simulink library "usask_segmented_TLM_lib"  (R2018a)
settings: Solver=VariableStepAuto  StartTime=0.0  StopTime=10.0  RelTol=1e-3
values from neighbouring files (symbols this model uses):
  beta = [1e-05 1.21547425008e-05 1.4773776526e-05 1.79571449437e-05 2.1826447284e-05 2.65294846443e-05 3.2245905453e-05 3.91940677485e-05 4.7639380104e-05 5.7904439806e-05 7.03813555493e-05 8.55467253557e-05 ... (60 elements, 1x60)]    [G_lookup.mat]    (also in H_lookup.mat)
  lambda_A = [0.333333333333 0.351351351351 0.369863013699 0.388888888889 0.408450704225 0.428571428571 0.449275362319 0.470588235294 0.492537313433 0.515151515152 0.538461538462 0.5625 ... (51 elements, 1x51)]    [H_lookup.mat]
  n = [6 3 2 1.5 1.2 1]    [G_lookup.mat]    (also in interpolate_G.m = lu_data.n)
  n1 = [0 16.6666666667 8.33333333333 5.55555555556 4.16666666667 3.33333333333]    [H_lookup.mat]    (also in interpolate_H.m = lu_data.n1)
  n2 = [0 16.6666666667 8.33333333333 5.55555555556 4.16666666667 3.33333333333]    [H_lookup.mat]    (also in interpolate_H.m = lu_data.n2)
  n3 = [3.16296285985 3.12622720794 3.08950324161 3.03556206993 2.98109456935 2.92539200093 2.86604767633 2.80095613668 2.7359041708 2.66771255902 2.60605912149 2.43399666463 ... (3060 elements, 60x51)]    [H_lookup.mat]    (also in interpolate_H.m = interp2(lu_data.phi_A,log10(lu_data.beta),lu_data.n3,phi,log)
  W1 = [0.817804106601 -0.379201060736 4.74543844452 -19.7629025979 31.2965927958 -16.3931724883 0.817756661365 -0.379072651507 4.74402355955 -19.7576226526 31.2889826509 -16.3894979768 ... (18360 elements, 1x6x60x51)]    [H_lookup.mat]    (also in interpolate_H.m = nan(size(n1)))
  W2 = [-0.0342032638777 0.250736765493 -2.89749565946 11.0980283604 -15.789942854 7.03898081697 -0.034202667139 0.250724810196 -2.89736972734 11.0975869151 -15.789368559 7.03873652617 ... (18360 elements, 1x6x60x51)]    [H_lookup.mat]    (also in interpolate_H.m = nan(size(n2)))
  W3 = H_DC3*n3/2    [interpolate_H.m]
undefined symbols (not defined in the file or in its folder): K, L, m_G, nu, rA, rB, rho, T, Zc_A, Zc_B
libraries: $bdroot x34
settings Model: Creator=tkw954  LastModifiedBy=tkw954

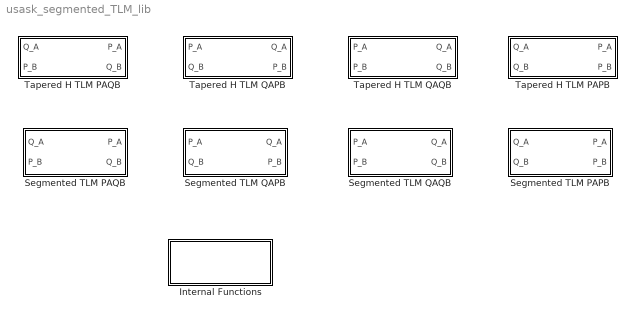
== system usask_segmented_TLM_lib ==
  Internal Functions : Subsystem
  Segmented TLM PAPB : Subsystem  mask{x_LU=100*[0 0.5 1], d_LU=12e-3*[1 0.8 1], K=1e6, nu=100e-6, rho=850}
      mask prompts: x_LU "Shape Lookup Lengths (m)"; d_LU "Shape Lookup Diameters (m)"; K "Oil Bulk Modulus (Pa)"; nu "Oil Viscosity (m^2/s)"; rho "Oil Density (kg/m^3)"
      mask init:
      | if numel(x_LU)~=numel(d_LU)
      |     error('size of x lookup table must be same as d lookup table')
      | end
      | 
      | 
      | dx = 120;
      | y = 30;
      | w_seg = 70;
      | %w_min=30;
      | %w_space=20;
      | h = 100;
      | 
      | x_LU=x_LU-x_LU(1);%ensure first point is 0
      | 
      | N=numel(x_LU)-1;%number of segments
      | 
      | %model parameters
      | 
      | c=sqrt(K/rho);
      | Zc=rho*c./(pi/4*d_LU.^2);
      | Zc_A=Zc(1);
      | Zc_B=Zc(end);
      | 
      | delta_x=diff(x_LU);
      | T=delta_x/c
      | 
      | lambda_A=d_LU(2:end)./d_LU(1:(end-1))
      | 
      | beta = ((nu*delta_x)./(c*(d_LU(1:(end-1))/2).^2)).*((lambda_A.^2+lambda_A+1).^2./(9*lambda_A.^3)) % Dissipation number (dimensionless)
      | 
      | % 
      | % %find and delete old blocks and lines
      | sys=gcb;
      | hcb=get_param(sys,'Handle');
      | hb=get(hcb,'blocks');
      | segment_name='segment';
      | idx_seg=find(strncmp(hb,segment_name,numel(segment_name)));%find segments
      | assignin('base','hb',hb)
      | assignin('base','hcb',hcb)
      | assignin('base','idx_seg',idx_seg)
      | 
      | for i=1:numel(idx_seg)
      |     delete_block(sprintf('%s/%s',sys, hb{idx_seg(i)}))
      | end
      | 
      | hlines=get(hcb,'lines');
      | for i=1:numel(hlines)
      |     delete_line(hlines(i).Handle)
      | end
      | 
      | for i=1:N
      |     pos = [dx*i y dx*i+w_seg y+h];
      |     add_block('usask_segmented_TLM_lib/Internal Functions/Tapered TLM Segment',sprintf('%s/%s_%d',sys,segment_name, i),'Position',pos);
      |       set_param(sprintf('%s/%s_%d',sys,segment_name, i),'beta',sprintf('beta(%d)',i));
      |           set_param(sprintf('%s/%s_%d',sys,segment_name, i),'T',sprintf('T(%d)',i));
      |           set_param(sprintf('%s/%s_%d',sys,segment_name, i),'lambda_A',sprintf('lambda_A(%d)',i));
      | 
      | 
      | end
      | % 
      | % 
      | 
      | add_line(sys,'Q_A/1','Boundary A/1','autorouting','on')
      | add_line(sys,'Boundary A/1','P_A/1','autorouting','on')
      | add_line(sys,'Q_B/1','Boundary B/1','autorouting','on')
      | add_line(sys,'Boundary B/1','P_B/1','autorouting','on')
      | 
      | add_line(sys,'Boundary A/2','segment_1/1','autorouting','on')
      | add_line(sys,'segment_1/1','Boundary A/2','autorouting','on')
      | 
      | add_line(sys,'Boundary B/2',sprintf('%s_%d/2',segment_name, N),'autorouting','on')
      | add_line(sys,sprintf('%s_%d/2',segment_name, N),'Boundary B/2','autorouting','on')
      | 
      | for i=1:(N-1)
      |     add_line(sys,sprintf('segment_%d/2',i),sprintf('segment_%d/1',i+1),'autorouting','on')
      |      add_line(sys,sprintf('segment_%d/1',i+1),sprintf('segment_%d/2',i),'autorouting','on')
      |    
      | end
      mask Display:
      | port_label('input', 1 , '\itq_A', 'texmode', 'on')
      | port_label('input', 2 , '\itq_B', 'texmode', 'on')
      | port_label('output', 1 , '\itp_A', 'texmode', 'on')
      | port_label('output', 2 , '\itp_B', 'texmode', 'on')
      | 
      | plot(x_LU,d_LU)
      | plot(x_LU,-d_LU)
  Segmented TLM PAQB : Subsystem  mask{x_LU=100*[0 0.5 1], d_LU=12e-3*[1 0.8 1], K=1e6, nu=100e-6, rho=850}
      mask prompts: x_LU "Shape Lookup Lengths (m)"; d_LU "Shape Lookup Diameters (m)"; K "Oil Bulk Modulus (Pa)"; nu "Oil Viscosity (m^2/s)"; rho "Oil Density (kg/m^3)"
      mask init:
      | if numel(x_LU)~=numel(d_LU)
      |     error('size of x lookup table must be same as d lookup table')
      | end
      | 
      | 
      | dx = 120;
      | y = 30;
      | w_seg = 70;
      | %w_min=30;
      | %w_space=20;
      | h = 100;
      | 
      | x_LU=x_LU-x_LU(1);%ensure first point is 0
      | 
      | N=numel(x_LU)-1;%number of segments
      | 
      | %model parameters
      | 
      | c=sqrt(K/rho);
      | Zc=rho*c./(pi/4*d_LU.^2);
      | Zc_A=Zc(1);
      | Zc_B=Zc(end);
      | 
      | delta_x=diff(x_LU);
      | T=delta_x/c
      | 
      | lambda_A=d_LU(2:end)./d_LU(1:(end-1))
      | 
      | beta = ((nu*delta_x)./(c*(d_LU(1:(end-1))/2).^2)).*((lambda_A.^2+lambda_A+1).^2./(9*lambda_A.^3)) % Dissipation number (dimensionless)
      | 
      | % 
      | % %find and delete old blocks and lines
      | sys=gcb;
      | hcb=get_param(sys,'Handle');
      | hb=get(hcb,'blocks');
      | segment_name='segment';
      | idx_seg=find(strncmp(hb,segment_name,numel(segment_name)));%find segments
      | assignin('base','hb',hb)
      | assignin('base','hcb',hcb)
      | assignin('base','idx_seg',idx_seg)
      | 
      | for i=1:numel(idx_seg)
      |     delete_block(sprintf('%s/%s',sys, hb{idx_seg(i)}))
      | end
      | 
      | hlines=get(hcb,'lines');
      | for i=1:numel(hlines)
      |     delete_line(hlines(i).Handle)
      | end
      | 
      | for i=1:N
      |     pos = [dx*i y dx*i+w_seg y+h];
      |     add_block('usask_segmented_TLM_lib/Internal Functions/Tapered TLM Segment',sprintf('%s/%s_%d',sys,segment_name, i),'Position',pos);
      |       set_param(sprintf('%s/%s_%d',sys,segment_name, i),'beta',sprintf('beta(%d)',i));
      |           set_param(sprintf('%s/%s_%d',sys,segment_name, i),'T',sprintf('T(%d)',i));
      |           set_param(sprintf('%s/%s_%d',sys,segment_name, i),'lambda_A',sprintf('lambda_A(%d)',i));
      | 
      | 
      | end
      | % 
      | % 
      | 
      | add_line(sys,'Q_A/1','Boundary A/1','autorouting','on')
      | add_line(sys,'Boundary A/1','P_A/1','autorouting','on')
      | add_line(sys,'P_B/1','Boundary B/1','autorouting','on')
      | add_line(sys,'Boundary B/1','Q_B/1','autorouting','on')
      | 
      | add_line(sys,'Boundary A/2','segment_1/1','autorouting','on')
      | add_line(sys,'segment_1/1','Boundary A/2','autorouting','on')
      | 
      | add_line(sys,'Boundary B/2',sprintf('%s_%d/2',segment_name, N),'autorouting','on')
      | add_line(sys,sprintf('%s_%d/2',segment_name, N),'Boundary B/2','autorouting','on')
      | 
      | for i=1:(N-1)
      |     add_line(sys,sprintf('segment_%d/2',i),sprintf('segment_%d/1',i+1),'autorouting','on')
      |      add_line(sys,sprintf('segment_%d/1',i+1),sprintf('segment_%d/2',i),'autorouting','on')
      |    
      | end
      mask Display:
      | port_label('input', 1 , '\itq_A', 'texmode', 'on')
      | port_label('input', 2 , '\itp_B', 'texmode', 'on')
      | port_label('output', 1 , '\itp_A', 'texmode', 'on')
      | port_label('output', 2 , '\itq_B', 'texmode', 'on')
      | 
      | plot(x_LU,d_LU)
      | plot(x_LU,-d_LU)
  Segmented TLM QAPB : Subsystem  mask{x_LU=100*[0 0.5 1], d_LU=12e-3*[1 0.8 1], K=1e9, nu=100e-6, rho=850}
      mask prompts: x_LU "Shape Lookup Lengths (m)"; d_LU "Shape Lookup Diameters (m)"; K "Oil Bulk Modulus (Pa)"; nu "Oil Viscosity (m^2/s)"; rho "Oil Density (kg/m^3)"
      mask init:
      | if numel(x_LU)~=numel(d_LU)
      |     error('size of x lookup table must be same as d lookup table')
      | end
      | 
      | 
      | dx = 120;
      | y = 30;
      | w_seg = 70;
      | %w_min=30;
      | %w_space=20;
      | h = 100;
      | 
      | x_LU=x_LU-x_LU(1);%ensure first point is 0
      | 
      | N=numel(x_LU)-1;%number of segments
      | 
      | %model parameters
      | 
      | c=sqrt(K/rho);
      | Zc=rho*c./(pi/4*d_LU.^2);
      | Zc_A=Zc(1);
      | Zc_B=Zc(end);
      | 
      | delta_x=diff(x_LU);
      | T=delta_x/c
      | 
      | lambda_A=d_LU(2:end)./d_LU(1:(end-1))
      | 
      | beta = ((nu*delta_x)./(c*(d_LU(1:(end-1))/2).^2)).*((lambda_A.^2+lambda_A+1).^2./(9*lambda_A.^3)) % Dissipation number (dimensionless)
      | 
      | % 
      | % %find and delete old blocks and lines
      | sys=gcb;
      | hcb=get_param(sys,'Handle');
      | hb=get(hcb,'blocks');
      | segment_name='segment';
      | idx_seg=find(strncmp(hb,segment_name,numel(segment_name)));%find segments
      | assignin('base','hb',hb)
      | assignin('base','hcb',hcb)
      | assignin('base','idx_seg',idx_seg)
      | 
      | for i=1:numel(idx_seg)
      |     delete_block(sprintf('%s/%s',sys, hb{idx_seg(i)}))
      | end
      | 
      | hlines=get(hcb,'lines');
      | for i=1:numel(hlines)
      |     delete_line(hlines(i).Handle)
      | end
      | 
      | for i=1:N
      |     pos = [dx*i y dx*i+w_seg y+h];
      |     add_block('usask_segmented_TLM_lib/Internal Functions/Tapered TLM Segment',sprintf('%s/%s_%d',sys,segment_name, i),'Position',pos);
      |       set_param(sprintf('%s/%s_%d',sys,segment_name, i),'beta',sprintf('beta(%d)',i));
      |           set_param(sprintf('%s/%s_%d',sys,segment_name, i),'T',sprintf('T(%d)',i));
      |           set_param(sprintf('%s/%s_%d',sys,segment_name, i),'lambda_A',sprintf('lambda_A(%d)',i));
      | 
      | 
      | end
      | % 
      | % 
      | 
      | add_line(sys,'P_A/1','Boundary A/1','autorouting','on')
      | add_line(sys,'Boundary A/1','Q_A/1','autorouting','on')
      | add_line(sys,'Q_B/1','Boundary B/1','autorouting','on')
      | add_line(sys,'Boundary B/1','P_B/1','autorouting','on')
      | 
      | add_line(sys,'Boundary A/2','segment_1/1','autorouting','on')
      | add_line(sys,'segment_1/1','Boundary A/2','autorouting','on')
      | 
      | add_line(sys,'Boundary B/2',sprintf('%s_%d/2',segment_name, N),'autorouting','on')
      | add_line(sys,sprintf('%s_%d/2',segment_name, N),'Boundary B/2','autorouting','on')
      | 
      | for i=1:(N-1)
      |     add_line(sys,sprintf('segment_%d/2',i),sprintf('segment_%d/1',i+1),'autorouting','on')
      |      add_line(sys,sprintf('segment_%d/1',i+1),sprintf('segment_%d/2',i),'autorouting','on')
      |    
      | end
      mask Display:
      | port_label('input', 1 , '\itp_A', 'texmode', 'on')
      | port_label('input', 2 , '\itq_B', 'texmode', 'on')
      | port_label('output', 1 , '\itq_A', 'texmode', 'on')
      | port_label('output', 2 , '\itp_B', 'texmode', 'on')
      | 
      | plot(x_LU,d_LU)
      | plot(x_LU,-d_LU)
  Segmented TLM QAQB : Subsystem  mask{x_LU=100*[0 0.5 1], d_LU=12e-3*[1 0.8 1], K=1e9, nu=100e-6, rho=850}
      mask prompts: x_LU "Shape Lookup Lengths (m)"; d_LU "Shape Lookup Diameters (m)"; K "Oil Bulk Modulus (Pa)"; nu "Oil Viscosity (m^2/s)"; rho "Oil Density (kg/m^3)"
      mask init:
      | if numel(x_LU)~=numel(d_LU)
      |     error('size of x lookup table must be same as d lookup table')
      | end
      | 
      | 
      | dx = 120;
      | y = 30;
      | w_seg = 70;
      | %w_min=30;
      | %w_space=20;
      | h = 100;
      | 
      | x_LU=x_LU-x_LU(1);%ensure first point is 0
      | 
      | lambda_A=d_LU(2:end)./d_LU(1:(end-1));
      | 
      | phi=(lambda_A-1)./(lambda_A+1);
      | 
      | phi_max=0.5;
      | 
      | while any(abs(phi)>phi_max)
      |     idx=find(abs(phi)>phi_max,1);
      |     d_LU=[d_LU(1:idx) (d_LU(idx)+d_LU(idx+1))/2 d_LU((idx+1):end)];
      |     x_LU=[x_LU(1:idx) (x_LU(idx)+x_LU(idx+1))/2 x_LU((idx+1):end)];
      |     lambda_A=d_LU(2:end)./d_LU(1:(end-1));
      | 
      |     phi=(lambda_A-1)./(lambda_A+1);
      | end
      | 
      | 
      | N=numel(x_LU)-1;%number of segments
      | 
      | %model parameters
      | 
      | c=sqrt(K/rho);
      | Zc=rho*c./(pi/4*d_LU.^2);
      | Zc_A=Zc(1);
      | Zc_B=Zc(end);
      | 
      | delta_x=diff(x_LU);
      | T=delta_x/c
      | 
      | 
      | 
      | beta = ((nu*delta_x)./(c*(d_LU(1:(end-1))/2).^2)).*((lambda_A.^2+lambda_A+1).^2./(9*lambda_A.^3)) % Dissipation number (dimensionless)
      | lambda_A
      | 
      | % 
      | % %find and delete old blocks and lines
      | sys=gcb;
      | hcb=get_param(sys,'Handle');
      | hb=get(hcb,'blocks');
      | segment_name='segment';
      | idx_seg=find(strncmp(hb,segment_name,numel(segment_name)));%find segments
      | assignin('base','hb',hb)
      | assignin('base','hcb',hcb)
      | assignin('base','idx_seg',idx_seg)
      | 
      | for i=1:numel(idx_seg)
      |     delete_block(sprintf('%s/%s',sys, hb{idx_seg(i)}))
      | end
      | 
      | hlines=get(hcb,'lines');
      | for i=1:numel(hlines)
      |     delete_line(hlines(i).Handle)
      | end
      | 
      | for i=1:N
      |     pos = [dx*i y dx*i+w_seg y+h];
      |     add_block('usask_segmented_TLM_lib/Internal Functions/Tapered TLM Segment',sprintf('%s/%s_%d',sys,segment_name, i),'Position',pos);
      |       set_param(sprintf('%s/%s_%d',sys,segment_name, i),'beta',sprintf('beta(%d)',i));
      |           set_param(sprintf('%s/%s_%d',sys,segment_name, i),'T',sprintf('T(%d)',i));
      |           set_param(sprintf('%s/%s_%d',sys,segment_name, i),'lambda_A',sprintf('lambda_A(%d)',i));
      | 
      | 
      | end
      | % 
      | % 
      | 
      | add_line(sys,'P_A/1','Boundary A/1','autorouting','on')
      | add_line(sys,'Boundary A/1','Q_A/1','autorouting','on')
      | add_line(sys,'P_B/1','Boundary B/1','autorouting','on')
      | add_line(sys,'Boundary B/1','Q_B/1','autorouting','on')
      | 
      | add_line(sys,'Boundary A/2','segment_1/1','autorouting','on')
      | add_line(sys,'segment_1/1','Boundary A/2','autorouting','on')
      | 
      | add_line(sys,'Boundary B/2',sprintf('%s_%d/2',segment_name, N),'autorouting','on')
      | add_line(sys,sprintf('%s_%d/2',segment_name, N),'Boundary B/2','autorouting','on')
      | 
      | for i=1:(N-1)
      |     add_line(sys,sprintf('segment_%d/2',i),sprintf('segment_%d/1',i+1),'autorouting','on')
      |      add_line(sys,sprintf('segment_%d/1',i+1),sprintf('segment_%d/2',i),'autorouting','on')
      |    
      | end
      mask Display:
      | port_label('input', 1 , '\itp_A', 'texmode', 'on')
      | port_label('input', 2 , '\itp_B', 'texmode', 'on')
      | port_label('output', 1 , '\itq_A', 'texmode', 'on')
      | port_label('output', 2 , '\itq_B', 'texmode', 'on')
      | 
      | plot(x_LU,d_LU)
      | plot(x_LU,-d_LU)
  Tapered H TLM PAPB : Subsystem  mask(Tapered Hydraulic Transmission Line (TLM)){D_A=rA*2, D_B=rB*2, L=L, K=K, nu=nu, rho=rho}
      mask prompts: D_A "Inlet Diameter (m)"; D_B "Outlet Diameter (m)"; L "Length (m)"; K "Oil Bulk Modulus (Pa)"; nu "Oil Viscosity (m^2/s)"; rho "Oil Density (kg/m^3)"
      mask help:
      | This model implements the transmission line model in Wiens and ven der Buhs (2018).
      |
      | This model assumes a rigid-walled tube with a linear taper in radius between the two ports. It assumes constant bulk modulus (no cavitation or entrained air effects) and includes frequency-dependent friction effects.
      |
      | Positive flows are directed into either port.
      |
      | This model also assumes zero initial conditions
      |
      | Reference:
      | Travis Wiens and Jeremy vsn der Buhs. Transmission Line Modelling of Laminar Liquid Wave Propagation in Tapered Tubes. In preparation.
      mask init:
      | % Check for positive params, report error if negative given
      | if D_A<0 || D_B<0 || L<0 || K<0 || nu<0 || rho<0
      |     error('Please ensure parameters are all positive')
      | end
      | 
      | r_A = D_A/2; % Inlet radius (m)
      | r_B = D_B/2; % Outlet radius (m)
      | 
      | c=sqrt(K/rho);% Local speed of sound (m/s)
      | lambda_A = r_B/r_A; % Taper ratio (dimensionless)
      | beta = ((nu*L)/(c*r_A^2))*((lambda_A^2+lambda_A+1)^2/(9*lambda_A^3)); % Dissipation number (dimensionless)
      | Zc_A=c*rho/(pi*r_A^2);
      | Zc_B=c*rho/(pi*r_B^2);
      | T=L/c; % Wave propagation time (s)
      mask DialogControl DescGroupVar Prompt: Tapered Hydraulic Transmission Line (TLM)
      mask Display:
      | port_label('input', 1 , '\itq_A', 'texmode', 'on')
      | port_label('input', 2 , '\itq_B', 'texmode', 'on')
      | port_label('output', 1 , '\itp_A', 'texmode', 'on')
      | port_label('output', 2 , '\itp_B', 'texmode', 'on')
  Tapered H TLM PAQB : Subsystem  mask(Tapered Hydraulic Transmission Line (TLM)){D_A=rA*2, D_B=rB*2, L=L, K=K, nu=nu, rho=rho}
      mask prompts: D_A "Inlet Diameter (m)"; D_B "Outlet Diameter (m)"; L "Length (m)"; K "Oil Bulk Modulus (Pa)"; nu "Oil Viscosity (m^2/s)"; rho "Oil Density (kg/m^3)"
      mask help:
      | This model implements the transmission line model in Wiens and ven der Buhs (2018).
      |
      | This model assumes a rigid-walled tube with a linear taper in radius between the two ports. It assumes constant bulk modulus (no cavitation or entrained air effects) and includes frequency-dependent friction effects.
      |
      | Positive flows are directed into either port.
      |
      | This model also assumes zero initial conditions
      |
      | Reference:
      | Travis Wiens and Jeremy vsn der Buhs. Transmission Line Modelling of Laminar Liquid Wave Propagation in Tapered Tubes. In preparation.
      mask init:
      | % Check for positive params, report error if negative given
      | if D_A<0 || D_B<0 || L<0 || K<0 || nu<0 || rho<0
      |     error('Please ensure parameters are all positive')
      | end
      | 
      | r_A = D_A/2; % Inlet radius (m)
      | r_B = D_B/2; % Outlet radius (m)
      | 
      | c=sqrt(K/rho);% Local speed of sound (m/s)
      | lambda_A = r_B/r_A; % Taper ratio (dimensionless)
      | beta = ((nu*L)/(c*r_A^2))*((lambda_A^2+lambda_A+1)^2/(9*lambda_A^3)); % Dissipation number (dimensionless)
      | Zc_A=c*rho/(pi*r_A^2);
      | Zc_B=c*rho/(pi*r_B^2);
      | T=L/c; % Wave propagation time (s)
      mask DialogControl DescGroupVar Prompt: Tapered Hydraulic Transmission Line (TLM)
      mask Display:
      | port_label('input', 1 , '\itq_A', 'texmode', 'on')
      | port_label('input', 2 , '\itp_B', 'texmode', 'on')
      | port_label('output', 1 , '\itp_A', 'texmode', 'on')
      | port_label('output', 2 , '\itq_B', 'texmode', 'on')
  Tapered H TLM QAPB : Subsystem  mask(Tapered Hydraulic Transmission Line (TLM)){D_A=rA*2, D_B=rB*2, L=L, K=K, nu=nu, rho=rho}
      mask prompts: D_A "Inlet Diameter (m)"; D_B "Outlet Diameter (m)"; L "Length (m)"; K "Oil Bulk Modulus (Pa)"; nu "Oil Viscosity (m^2/s)"; rho "Oil Density (kg/m^3)"
      mask help:
      | This model implements the transmission line model in Wiens and ven der Buhs (2018).
      |
      | This model assumes a rigid-walled tube with a linear taper in radius between the two ports. It assumes constant bulk modulus (no cavitation or entrained air effects) and includes frequency-dependent friction effects.
      |
      | Positive flows are directed into either port.
      |
      | This model also assumes zero initial conditions
      |
      | Reference:
      | Travis Wiens and Jeremy vsn der Buhs. Transmission Line Modelling of Laminar Liquid Wave Propagation in Tapered Tubes. In preparation.
      mask init: same as usask_segmented_TLM_lib/Tapered H TLM PAPB
      mask DialogControl DescGroupVar Prompt: Tapered Hydraulic Transmission Line (TLM)
      mask Display:
      | port_label('input', 1 , '\itp_A', 'texmode', 'on')
      | port_label('input', 2 , '\itq_B', 'texmode', 'on')
      | port_label('output', 1 , '\itq_A', 'texmode', 'on')
      | port_label('output', 2 , '\itp_B', 'texmode', 'on')
  Tapered H TLM QAQB : Subsystem  mask(Tapered Hydraulic Transmission Line (TLM)){D_A=rA*2, D_B=rB*2, L=L, K=K, nu=nu, rho=rho}
      mask prompts: D_A "Inlet Diameter (m)"; D_B "Outlet Diameter (m)"; L "Length (m)"; K "Oil Bulk Modulus (Pa)"; nu "Oil Viscosity (m^2/s)"; rho "Oil Density (kg/m^3)"
      mask help:
      | This model implements the transmission line model in Wiens and ven der Buhs (2018).
      |
      | This model assumes a rigid-walled tube with a linear taper in radius between the two ports. It assumes constant bulk modulus (no cavitation or entrained air effects) and includes frequency-dependent friction effects.
      |
      | Positive flows are directed into either port.
      |
      | This model also assumes zero initial conditions
      |
      | Reference:
      | Travis Wiens and Jeremy vsn der Buhs. Transmission Line Modelling of Laminar Liquid Wave Propagation in Tapered Tubes. In preparation.
      mask init: same as usask_segmented_TLM_lib/Tapered H TLM PAQB
      mask DialogControl DescGroupVar Prompt: Tapered Hydraulic Transmission Line (TLM)
      mask Display:
      | port_label('input', 1 , '\itp_A', 'texmode', 'on')
      | port_label('input', 2 , '\itp_B', 'texmode', 'on')
      | port_label('output', 1 , '\itq_A', 'texmode', 'on')
      | port_label('output', 2 , '\itq_B', 'texmode', 'on')

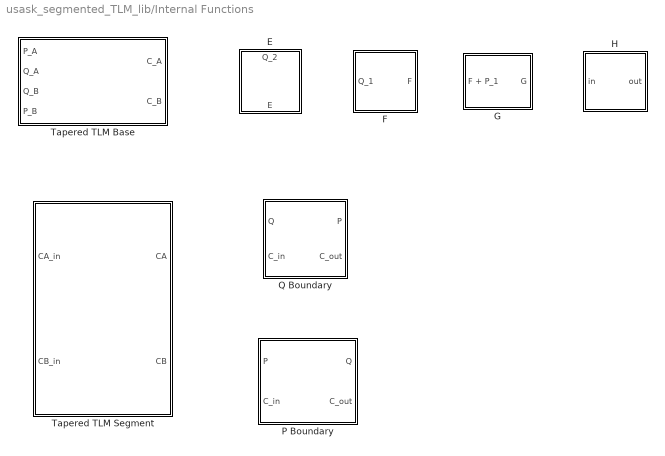
== system usask_segmented_TLM_lib/Internal Functions ==
  E : Subsystem
      mask Display: disp('\fontname{Times New Roman}\fontsize{30}\itE', 'texmode', 'on')
  F : Subsystem  mask{Zc=Zc_A}
      mask Display: disp('\fontname{Times New Roman}\fontsize{30}\itF', 'texmode', 'on')
  G : Subsystem  mask{lambda=lambda_A, beta=beta, T=T}
      mask init:
      | [m_G, n] = interpolate_G(lambda,beta);
      | 
      | lambda2=1/lambda;
      | R_Zc=24*beta/(1+lambda2+lambda2^2);
      | H_DC=(R_Zc+1/lambda2^2-1)./(R_Zc+1/lambda2^2+1);
      mask Display: disp('\fontname{Times New Roman}\fontsize{30}\itG', 'texmode', 'on')
  H : Subsystem  mask{lambda=lambda_A, beta=beta, T=T}
      mask init:
      | [W1,W2,W3,n1,n2,n3] = interpolate_H(lambda,beta);
      mask Display: disp('\fontname{Times New Roman}\fontsize{30}\itH', 'texmode', 'on')
  P Boundary : Subsystem  mask{Zc=Zc_B}
  Q Boundary : Subsystem  mask{Zc=Zc_A}
  Tapered TLM Base : Subsystem  mask(Tapered Hydraulic Transmission Line (TLM)){Zc_A=Zc_A, Zc_B=Zc_B, beta=beta, T=T, lambda_A=lambda_A}
      mask help:
      | This model implements the transmission line model in Wiens and ven der Buhs (2018).
      |
      | This model assumes laminar flow in a rigid-walled tube with a linear taper in radius between the two ports. It assumes constant bulk modulus (no cavitation or entrined air effects) and includes frequency-dependent friction effects.
      |
      | Positive flows are directed into either port.
      |
      | This model also assumes zero initial conditions
      |
      | Reference:
      | Travis Wiens and Jeremy vsn der Buhs. In Improved Transmission Line Model for Dynamic Laminar Flow Through Tapered Tubes. Proceedings of the Bath/ASME Symposium on Fluid Power and Motion Control, Bath, 2018
      mask init:
      | lambda_B=1/lambda_A;
      mask DialogControl DescGroupVar Prompt: Tapered Hydraulic Transmission Line (TLM)
  Tapered TLM Segment : Subsystem  mask{lambda_A=lambda_A(1), beta=beta(1), T=T(1)}
      mask init:
      | lambda_B=1/lambda_A;

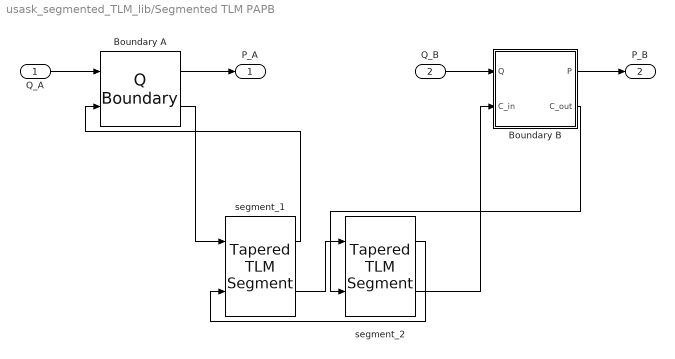
== system usask_segmented_TLM_lib/Segmented TLM PAPB ==
  Q_A : Inport
  Q_B : Inport  Port=2
  Boundary A : $bdroot/Internal Functions/Q Boundary  Zc=Zc_A
  Boundary B : Subsystem  mask{Zc=Zc_B}
  segment_1 : $bdroot/Internal Functions/Tapered TLM Segment  lambda_A=lambda_A(1)  beta=beta(1)  T=T(1)
  segment_2 : $bdroot/Internal Functions/Tapered TLM Segment  lambda_A=lambda_A(2)  beta=beta(2)  T=T(2)
  P_A : Outport
  P_B : Outport  Port=2
  wires:
  Q_A/1 -> Boundary A/1
  Boundary A/1 -> P_A/1
  Q_B/1 -> Boundary B/1(Q)
  Boundary B/1(P) -> P_B/1
  Boundary A/2 -> segment_1/1
  segment_1/1 -> Boundary A/2
  Boundary B/2(C_out) -> segment_2/2
  segment_2/2 -> Boundary B/2(C_in)
  segment_1/2 -> segment_2/1
  segment_2/1 -> segment_1/2

== system usask_segmented_TLM_lib/Segmented TLM PAQB ==
  Q_A : Inport
  P_B : Inport  Port=2
  Boundary A : $bdroot/Internal Functions/Q Boundary  Zc=Zc_A
  Boundary B : $bdroot/Internal Functions/P Boundary  Zc=Zc_B
  segment_1 : $bdroot/Internal Functions/Tapered TLM Segment  lambda_A=lambda_A(1)  beta=beta(1)  T=T(1)
  segment_2 : $bdroot/Internal Functions/Tapered TLM Segment  lambda_A=lambda_A(2)  beta=beta(2)  T=T(2)
  P_A : Outport
  Q_B : Outport  Port=2
  wires:
  Q_A/1 -> Boundary A/1
  Boundary A/1 -> P_A/1
  P_B/1 -> Boundary B/1
  Boundary B/1 -> Q_B/1
  Boundary A/2 -> segment_1/1
  segment_1/1 -> Boundary A/2
  Boundary B/2 -> segment_2/2
  segment_2/2 -> Boundary B/2
  segment_1/2 -> segment_2/1
  segment_2/1 -> segment_1/2

== system usask_segmented_TLM_lib/Segmented TLM QAPB ==
  P_A : Inport
  Q_B : Inport  Port=2
  Boundary A : $bdroot/Internal Functions/P Boundary  Zc=Zc_A
  Boundary B : $bdroot/Internal Functions/Q Boundary  Zc=Zc_B
  segment_1 : $bdroot/Internal Functions/Tapered TLM Segment  lambda_A=lambda_A(1)  beta=beta(1)  T=T(1)
  segment_2 : $bdroot/Internal Functions/Tapered TLM Segment  lambda_A=lambda_A(2)  beta=beta(2)  T=T(2)
  Q_A : Outport
  P_B : Outport  Port=2
  wires:
  P_A/1 -> Boundary A/1
  Boundary A/1 -> Q_A/1
  Q_B/1 -> Boundary B/1
  Boundary B/1 -> P_B/1
  Boundary A/2 -> segment_1/1
  segment_1/1 -> Boundary A/2
  Boundary B/2 -> segment_2/2
  segment_2/2 -> Boundary B/2
  segment_1/2 -> segment_2/1
  segment_2/1 -> segment_1/2

== system usask_segmented_TLM_lib/Segmented TLM QAQB ==
  P_A : Inport
  P_B : Inport  Port=2
  Boundary A : $bdroot/Internal Functions/P Boundary  Zc=Zc_A
  Boundary B : $bdroot/Internal Functions/P Boundary  Zc=Zc_B
  segment_1 : $bdroot/Internal Functions/Tapered TLM Segment  lambda_A=lambda_A(1)  beta=beta(1)  T=T(1)
  segment_2 : $bdroot/Internal Functions/Tapered TLM Segment  lambda_A=lambda_A(2)  beta=beta(2)  T=T(2)
  Q_A : Outport
  Q_B : Outport  Port=2
  wires:
  P_A/1 -> Boundary A/1
  Boundary A/1 -> Q_A/1
  P_B/1 -> Boundary B/1
  Boundary B/1 -> Q_B/1
  Boundary A/2 -> segment_1/1
  segment_1/1 -> Boundary A/2
  Boundary B/2 -> segment_2/2
  segment_2/2 -> Boundary B/2
  segment_1/2 -> segment_2/1
  segment_2/1 -> segment_1/2

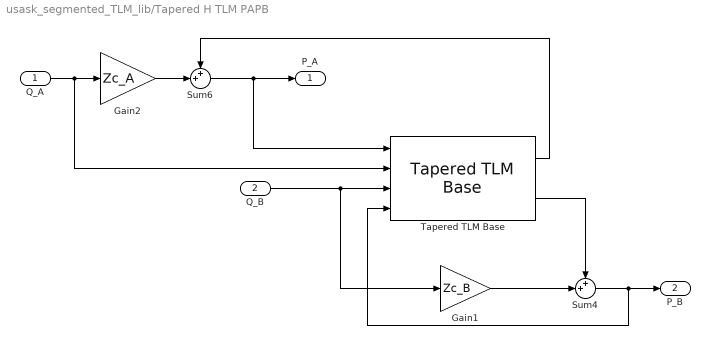
== system usask_segmented_TLM_lib/Tapered H TLM PAPB ==
  Q_A : Inport
  Q_B : Inport  Port=2
  Gain1 : Gain  Gain=Zc_B
  Gain2 : Gain  Gain=Zc_A
  Sum4 : Sum  Inputs=++|
  Sum6 : Sum  Inputs=++|
  Tapered TLM Base : $bdroot/Internal Functions/Tapered TLM Base  Zc_A=Zc_A  Zc_B=Zc_B  beta=beta  T=T  lambda_A=lambda_A
  P_A : Outport
  P_B : Outport  Port=2
  wires:
  Q_B/1 -> Gain1/1, Tapered TLM Base/3
  Tapered TLM Base/2 -> Sum4/1
  Gain1/1 -> Sum4/2
  Sum4/1 -> P_B/1, Tapered TLM Base/4
  Sum6/1 -> Tapered TLM Base/1, P_A/1
  Gain2/1 -> Sum6/2
  Tapered TLM Base/1 -> Sum6/1
  Q_A/1 -> Tapered TLM Base/2, Gain2/1

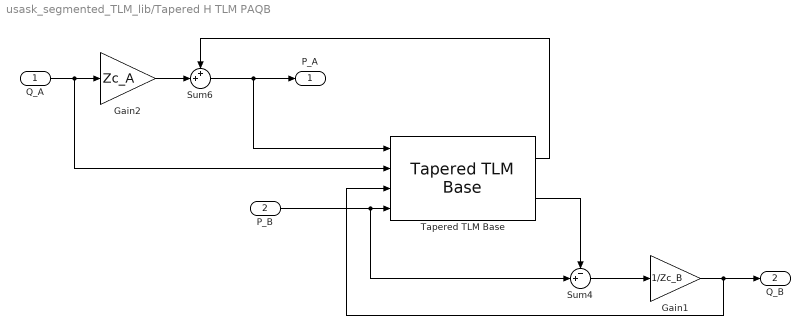
== system usask_segmented_TLM_lib/Tapered H TLM PAQB ==
  Q_A : Inport
  P_B : Inport  Port=2
  Gain1 : Gain  Gain=1/Zc_B
  Gain2 : Gain  Gain=Zc_A
  Sum4 : Sum  Inputs=-+|
  Sum6 : Sum  Inputs=++|
  Tapered TLM Base : $bdroot/Internal Functions/Tapered TLM Base  Zc_A=Zc_A  Zc_B=Zc_B  beta=beta  T=T  lambda_A=lambda_A
  P_A : Outport
  Q_B : Outport  Port=2
  wires:
  Q_A/1 -> Tapered TLM Base/2, Gain2/1
  Gain2/1 -> Sum6/2
  Sum6/1 -> Tapered TLM Base/1, P_A/1
  P_B/1 -> Tapered TLM Base/4, Sum4/2
  Tapered TLM Base/1 -> Sum6/1
  Tapered TLM Base/2 -> Sum4/1
  Sum4/1 -> Gain1/1
  Gain1/1 -> Tapered TLM Base/3, Q_B/1

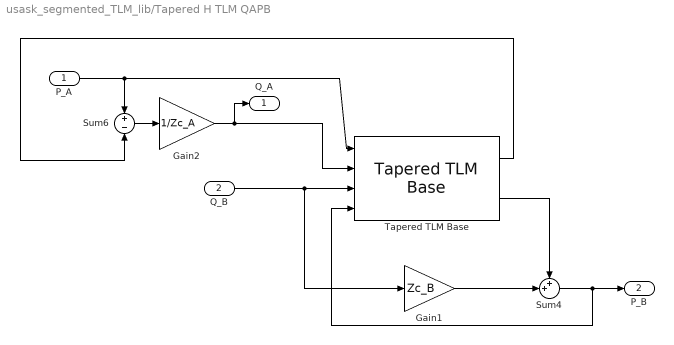
== system usask_segmented_TLM_lib/Tapered H TLM QAPB ==
  P_A : Inport
  Q_B : Inport  Port=2
  Gain1 : Gain  Gain=Zc_B
  Gain2 : Gain  Gain=1/Zc_A
  Sum4 : Sum  Inputs=++|
  Sum6 : Sum  Inputs=+|-
  Tapered TLM Base : $bdroot/Internal Functions/Tapered TLM Base  Zc_A=Zc_A  Zc_B=Zc_B  beta=beta  T=T  lambda_A=lambda_A
  Q_A : Outport
  P_B : Outport  Port=2
  wires:
  P_A/1 -> Sum6/1, Tapered TLM Base/1
  Tapered TLM Base/1 -> Sum6/2
  Gain2/1 -> Q_A/1, Tapered TLM Base/2
  Sum6/1 -> Gain2/1
  Q_B/1 -> Gain1/1, Tapered TLM Base/3
  Tapered TLM Base/2 -> Sum4/1
  Gain1/1 -> Sum4/2
  Sum4/1 -> P_B/1, Tapered TLM Base/4

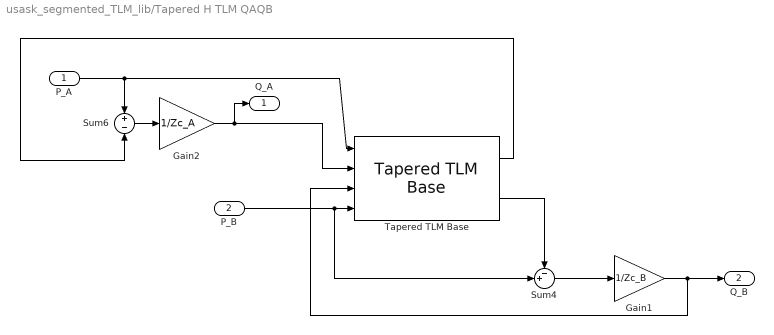
== system usask_segmented_TLM_lib/Tapered H TLM QAQB ==
  P_A : Inport
  P_B : Inport  Port=2
  Gain1 : Gain  Gain=1/Zc_B
  Gain2 : Gain  Gain=1/Zc_A
  Sum4 : Sum  Inputs=-+|
  Sum6 : Sum  Inputs=+|-
  Tapered TLM Base : $bdroot/Internal Functions/Tapered TLM Base  Zc_A=Zc_A  Zc_B=Zc_B  beta=beta  T=T  lambda_A=lambda_A
  Q_A : Outport
  Q_B : Outport  Port=2
  wires:
  P_B/1 -> Tapered TLM Base/4, Sum4/2
  Tapered TLM Base/2 -> Sum4/1
  Sum4/1 -> Gain1/1
  Gain1/1 -> Tapered TLM Base/3, Q_B/1
  Sum6/1 -> Gain2/1
  Tapered TLM Base/1 -> Sum6/2
  P_A/1 -> Tapered TLM Base/1, Sum6/1
  Gain2/1 -> Tapered TLM Base/2, Q_A/1

== system usask_segmented_TLM_lib/Internal Functions/E ==
  Q_2 : Inport
  Constant : Constant  Value=0
  Terminator1 : Terminator
  E : Outport
  wires:
  Q_2/1 -> Terminator1/1
  Constant/1 -> E/1

== system usask_segmented_TLM_lib/Internal Functions/F ==
  Q_1 : Inport
  Gain1 : Gain  Gain=Zc
  F : Outport
  wires:
  Q_1/1 -> Gain1/1
  Gain1/1 -> F/1

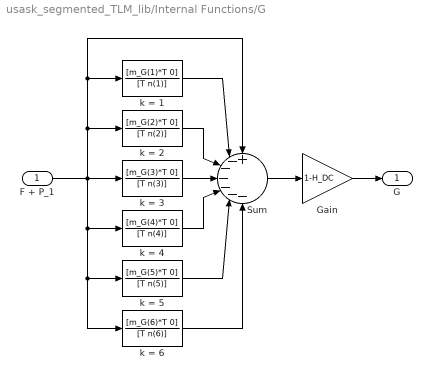
== system usask_segmented_TLM_lib/Internal Functions/G ==
  F + P_1 : Inport
  Gain : Gain  Gain=1-H_DC
  Sum : Sum  Inputs=+------
  k = 1 : TransferFcn  Numerator=[m_G(1)*T 0]  Denominator=[T n(1)]
  k = 2 : TransferFcn  Numerator=[m_G(2)*T 0]  Denominator=[T n(2)]
  k = 3 : TransferFcn  Numerator=[m_G(3)*T 0]  Denominator=[T n(3)]
  k = 4 : TransferFcn  Numerator=[m_G(4)*T 0]  Denominator=[T n(4)]
  k = 5 : TransferFcn  Numerator=[m_G(5)*T 0]  Denominator=[T n(5)]
  k = 6 : TransferFcn  Numerator=[m_G(6)*T 0]  Denominator=[T n(6)]
  G : Outport
  wires:
  Sum/1 -> Gain/1
  F + P_1/1 -> k = 4/1, k = 6/1, k = 5/1, k = 1/1, Sum/1, k = 2/1, k = 3/1
  k = 3/1 -> Sum/4
  k = 1/1 -> Sum/2
  k = 2/1 -> Sum/3
  k = 4/1 -> Sum/5
  k = 5/1 -> Sum/6
  k = 6/1 -> Sum/7
  Gain/1 -> G/1

== system usask_segmented_TLM_lib/Internal Functions/H ==
  in : Inport
  Add : Sum  Inputs=+++
  Part 1 : Subsystem  mask{W=W1, n=n1}
  Part 2 : Subsystem  mask{W=W2, n=n2}
  Part 3 : Subsystem  mask{W=W3, n=n3}
  Transport Delay1 : TransportDelay  DelayTime=2*T  BufferSize=2048
  Transport Delay2 : TransportDelay  DelayTime=2*T  BufferSize=2048
  out : Outport
  wires:
  in/1 -> Transport Delay1/1, Part 1/1(In1)
  Part 1/1(Out1) -> Add/1
  Transport Delay1/1 -> Transport Delay2/1, Part 2/1(In1)
  Part 2/1(Out1) -> Add/2
  Add/1 -> out/1
  Part 3/1(Out1) -> Add/3
  Transport Delay2/1 -> Part 3/1(In1)

== system usask_segmented_TLM_lib/Internal Functions/P Boundary ==
  P : Inport
  C_in : Inport  Port=2
  FB : $bdroot/Internal Functions/F  Zc=Zc
  Gain1 : Gain  Gain=1/Zc
  Sum3 : Sum  Inputs=|++
  Sum4 : Sum  Inputs=|+-
  Q : Outport
  C_out : Outport  Port=2
  wires:
  Gain1/1 -> Q/1, FB/1
  P/1 -> Sum3/2, Sum4/1
  FB/1 -> Sum3/1
  Sum4/1 -> Gain1/1
  C_in/1 -> Sum4/2
  Sum3/1 -> C_out/1

== system usask_segmented_TLM_lib/Internal Functions/Q Boundary ==
  Q : Inport
  C_in : Inport  Port=2
  FA : $bdroot/Internal Functions/F  Zc=Zc
  Gain2 : Gain  Gain=Zc
  Sum : Sum  Inputs=++|
  Sum6 : Sum  Inputs=|++
  P : Outport
  C_out : Outport  Port=2
  wires:
  Gain2/1 -> Sum6/1
  Q/1 -> Gain2/1, FA/1
  FA/1 -> Sum/1
  Sum/1 -> C_out/1
  Sum6/1 -> P/1, Sum/2
  C_in/1 -> Sum6/2

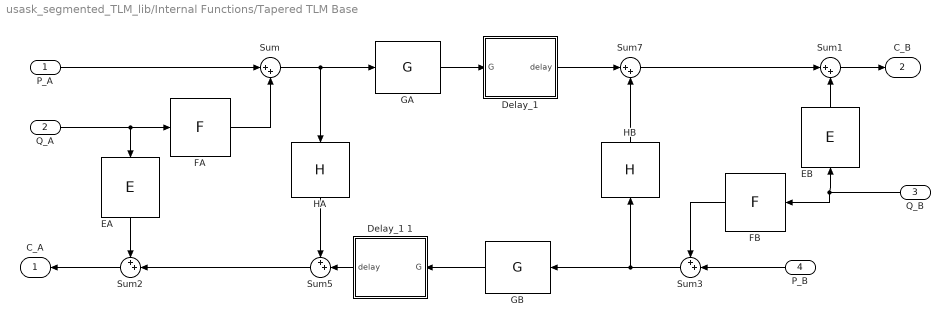
== system usask_segmented_TLM_lib/Internal Functions/Tapered TLM Base ==
  P_A : Inport
  Q_A : Inport  Port=2
  Q_B : Inport  Port=3
  P_B : Inport  Port=4
  "Delay_1 " : Subsystem  mask{T=T}
      mask prompts: T "delay time"
      mask Display: disp('\fontname{Times New Roman}\ite^{-j\omegaT}', 'texmode', 'on')
  Delay_1 1 : Subsystem  mask{T=T}
      mask prompts: T "delay time"
      mask Display: disp('\fontname{Times New Roman}\ite^{-j\omegaT}', 'texmode', 'on')
  EA : $bdroot/Internal Functions/E  SystemSampleTime=-1
  EB : $bdroot/Internal Functions/E  SystemSampleTime=-1
  FA : $bdroot/Internal Functions/F  Zc=Zc_A
  FB : $bdroot/Internal Functions/F  Zc=Zc_B
  GA : $bdroot/Internal Functions/G  lambda=lambda_A  beta=beta  T=T
  GB : $bdroot/Internal Functions/G  lambda=lambda_B  beta=beta  T=T
  HA : $bdroot/Internal Functions/H  lambda=lambda_A  beta=beta  T=T
  HB : $bdroot/Internal Functions/H  lambda=lambda_B  beta=beta  T=T
  Sum : Sum  Inputs=|++
  Sum1 : Sum  Inputs=|++
  Sum2 : Sum  Inputs=++|
  Sum3 : Sum  Inputs=++|
  Sum5 : Sum  Inputs=++|
  Sum7 : Sum  Inputs=|++
  C_A : Outport
  " C_B" : Outport  Port=2
  wires:
  GB/1 -> Delay_1 1/1(G)
  Q_A/1 -> FA/1, EA/1
  FB/1 -> Sum3/1
  Sum5/1 -> Sum2/2
  FA/1 -> Sum/2
  P_B/1 -> Sum3/2
  EB/1 -> Sum1/2
  GA/1 -> "Delay_1 "/1(G)
  Sum1/1 -> " C_B"/1
  Sum3/1 -> GB/1, HB/1
  Sum7/1 -> Sum1/1
  HB/1 -> Sum7/2
  Delay_1 1/1(delay) -> Sum5/2
  EA/1 -> Sum2/1
  Sum2/1 -> C_A/1
  Sum/1 -> GA/1, HA/1
  P_A/1 -> Sum/1
  HA/1 -> Sum5/1
  "Delay_1 "/1(delay) -> Sum7/1
  Q_B/1 -> FB/1, EB/1

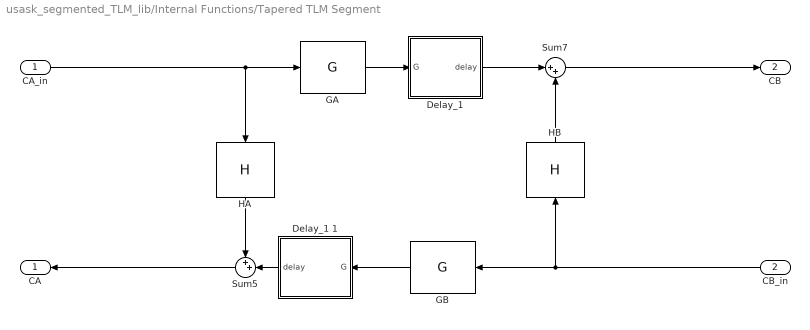
== system usask_segmented_TLM_lib/Internal Functions/Tapered TLM Segment ==
  CA_in : Inport
  CB_in : Inport  Port=2
  "Delay_1 " : Subsystem  mask{T=T}
      mask prompts: T "delay time"
      mask Display: disp('\fontname{Times New Roman}\ite^{-j\omegaT}', 'texmode', 'on')
  Delay_1 1 : Subsystem  mask{T=T}
      mask prompts: T "delay time"
      mask Display: disp('\fontname{Times New Roman}\ite^{-j\omegaT}', 'texmode', 'on')
  GA : $bdroot/Internal Functions/G  lambda=lambda_A  beta=beta  T=T
  GB : $bdroot/Internal Functions/G  lambda=lambda_B  beta=beta  T=T
  HA : $bdroot/Internal Functions/H  lambda=lambda_A  beta=beta  T=T
  HB : $bdroot/Internal Functions/H  lambda=lambda_B  beta=beta  T=T
  Sum5 : Sum  Inputs=++|
  Sum7 : Sum  Inputs=|++
  CA : Outport
  CB : Outport  Port=2
  wires:
  CA_in/1 -> HA/1, GA/1
  HB/1 -> Sum7/2
  GB/1 -> Delay_1 1/1(G)
  Delay_1 1/1(delay) -> Sum5/2
  "Delay_1 "/1(delay) -> Sum7/1
  GA/1 -> "Delay_1 "/1(G)
  HA/1 -> Sum5/1
  CB_in/1 -> HB/1, GB/1
  Sum7/1 -> CB/1
  Sum5/1 -> CA/1

== system usask_segmented_TLM_lib/Segmented TLM PAPB/Boundary B ==
  Q : Inport
  C_in : Inport  Port=2
  FA : $bdroot/Internal Functions/F  Zc=Zc
  Gain2 : Gain  Gain=Zc
  Sum : Sum  Inputs=++|
  Sum6 : Sum  Inputs=|++
  P : Outport
  C_out : Outport  Port=2
  wires:
  C_in/1 -> Sum6/2
  Sum6/1 -> Sum/2, P/1
  Sum/1 -> C_out/1
  FA/1 -> Sum/1
  Q/1 -> FA/1, Gain2/1
  Gain2/1 -> Sum6/1

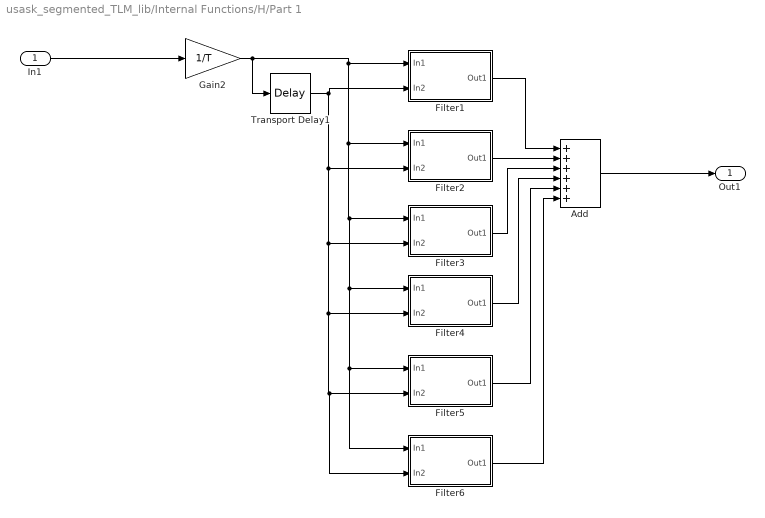
== system usask_segmented_TLM_lib/Internal Functions/H/Part 1 ==
  In1 : Inport
  Add : Sum  Inputs=++++++
  Filter1 : Subsystem  mask{W=W(1), n=n(1)}
      mask prompts: W "Wi"; n "ni"
  Filter2 : Subsystem  mask{W=W(2), n=n(2)}
      mask prompts: W "Wi"; n "ni"
  Filter3 : Subsystem  mask{W=W(3), n=n(3)}
      mask prompts: W "Wi"; n "ni"
  Filter4 : Subsystem  mask{W=W(4), n=n(4)}
      mask prompts: W "Wi"; n "ni"
  Filter5 : Subsystem  mask{W=W(5), n=n(5)}
      mask prompts: W "Wi"; n "ni"
  Filter6 : Subsystem  mask{W=W(6), n=n(6)}
      mask prompts: W "Wi"; n "ni"
  Gain2 : Gain  Gain=1/T
  Transport Delay1 : TransportDelay  DelayTime=2*T  BufferSize=2048
  Out1 : Outport
  wires:
  Filter6/1(Out1) -> Add/6
  Filter5/1(Out1) -> Add/5
  Filter4/1(Out1) -> Add/4
  Filter3/1(Out1) -> Add/3
  Filter2/1(Out1) -> Add/2
  Transport Delay1/1 -> Filter1/2(In2), Filter2/2(In2), Filter3/2(In2), Filter4/2(In2), Filter5/2(In2), Filter6/2(In2)
  Filter1/1(Out1) -> Add/1
  Gain2/1 -> Filter1/1(In1), Filter2/1(In1), Filter3/1(In1), Filter4/1(In1), Filter5/1(In1), Filter6/1(In1), Transport Delay1/1
  Add/1 -> Out1/1
  In1/1 -> Gain2/1

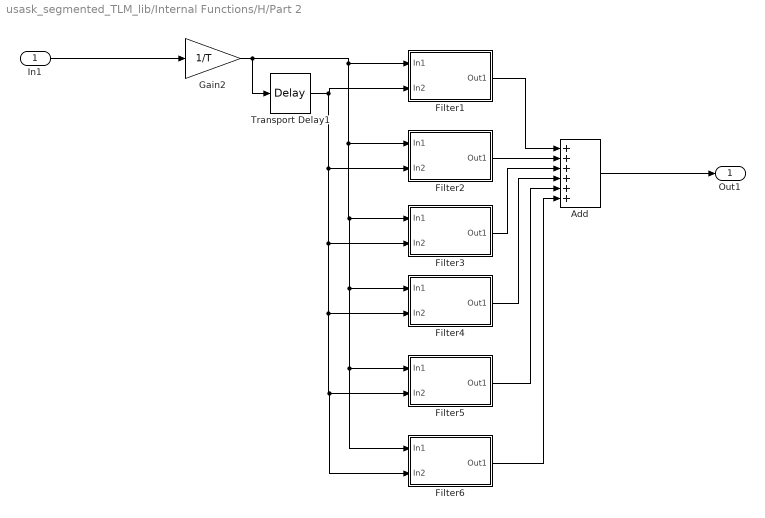
== system usask_segmented_TLM_lib/Internal Functions/H/Part 2 ==
  In1 : Inport
  Add : Sum  Inputs=++++++
  Filter1 : Subsystem  mask{W=W(1), n=n(1)}
      mask prompts: W "Wi"; n "ni"
  Filter2 : Subsystem  mask{W=W(2), n=n(2)}
      mask prompts: W "Wi"; n "ni"
  Filter3 : Subsystem  mask{W=W(3), n=n(3)}
      mask prompts: W "Wi"; n "ni"
  Filter4 : Subsystem  mask{W=W(4), n=n(4)}
      mask prompts: W "Wi"; n "ni"
  Filter5 : Subsystem  mask{W=W(5), n=n(5)}
      mask prompts: W "Wi"; n "ni"
  Filter6 : Subsystem  mask{W=W(6), n=n(6)}
      mask prompts: W "Wi"; n "ni"
  Gain2 : Gain  Gain=1/T
  Transport Delay1 : TransportDelay  DelayTime=2*T  BufferSize=2048
  Out1 : Outport
  wires:
  Filter6/1(Out1) -> Add/6
  Filter5/1(Out1) -> Add/5
  Filter4/1(Out1) -> Add/4
  Filter3/1(Out1) -> Add/3
  Filter2/1(Out1) -> Add/2
  Transport Delay1/1 -> Filter1/2(In2), Filter2/2(In2), Filter3/2(In2), Filter4/2(In2), Filter5/2(In2), Filter6/2(In2)
  Filter1/1(Out1) -> Add/1
  Gain2/1 -> Filter1/1(In1), Filter2/1(In1), Filter3/1(In1), Filter4/1(In1), Filter5/1(In1), Filter6/1(In1), Transport Delay1/1
  Add/1 -> Out1/1
  In1/1 -> Gain2/1

== system usask_segmented_TLM_lib/Internal Functions/H/Part 3 ==
  In1 : Inport
  Gain2 : Gain  Gain=1/T
  Transfer Fcn : TransferFcn  Numerator=[W(1)]  Denominator=[1 n(1)/(2*T)]
  Out1 : Outport
  wires:
  Gain2/1 -> Transfer Fcn/1
  In1/1 -> Gain2/1
  Transfer Fcn/1 -> Out1/1

== system usask_segmented_TLM_lib/Internal Functions/Tapered TLM Base/Delay_1  ==
  G : Inport
  Transport Delay : TransportDelay  DelayTime=T
  delay : Outport
  wires:
  G/1 -> Transport Delay/1
  Transport Delay/1 -> delay/1

== system usask_segmented_TLM_lib/Internal Functions/Tapered TLM Base/Delay_1 1 ==
  G : Inport
  Transport Delay : TransportDelay  DelayTime=T
  delay : Outport
  wires:
  G/1 -> Transport Delay/1
  Transport Delay/1 -> delay/1

== system usask_segmented_TLM_lib/Internal Functions/Tapered TLM Segment/Delay_1  ==
  G : Inport
  Transport Delay : TransportDelay  DelayTime=T
  delay : Outport
  wires:
  Transport Delay/1 -> delay/1
  G/1 -> Transport Delay/1

== system usask_segmented_TLM_lib/Internal Functions/Tapered TLM Segment/Delay_1 1 ==
  G : Inport
  Transport Delay : TransportDelay  DelayTime=T
  delay : Outport
  wires:
  Transport Delay/1 -> delay/1
  G/1 -> Transport Delay/1

== system usask_segmented_TLM_lib/Internal Functions/H/Part 1/Filter1 ==
  In1 : Inport
  In2 : Inport  Port=2
  Add1 : Sum  Inputs=+-
  Gain1 : Gain  Gain=exp(-n)
  Transfer Fcn : TransferFcn  Numerator=[W]  Denominator=[1 n/(2*T)]
  Transfer Fcn1 : TransferFcn  Numerator=[W]  Denominator=[1 n/(2*T)]
  Out1 : Outport
  wires:
  In2/1 -> Transfer Fcn1/1
  Gain1/1 -> Add1/2
  In1/1 -> Transfer Fcn/1
  Transfer Fcn/1 -> Add1/1
  Transfer Fcn1/1 -> Gain1/1
  Add1/1 -> Out1/1

== system usask_segmented_TLM_lib/Internal Functions/H/Part 1/Filter2 ==
  In1 : Inport
  In2 : Inport  Port=2
  Add1 : Sum  Inputs=+-
  Gain1 : Gain  Gain=exp(-n)
  Transfer Fcn : TransferFcn  Numerator=[W]  Denominator=[1 n/(2*T)]
  Transfer Fcn1 : TransferFcn  Numerator=[W]  Denominator=[1 n/(2*T)]
  Out1 : Outport
  wires:
  Add1/1 -> Out1/1
  Transfer Fcn1/1 -> Gain1/1
  Transfer Fcn/1 -> Add1/1
  In1/1 -> Transfer Fcn/1
  Gain1/1 -> Add1/2
  In2/1 -> Transfer Fcn1/1

== system usask_segmented_TLM_lib/Internal Functions/H/Part 1/Filter3 ==
  In1 : Inport
  In2 : Inport  Port=2
  Add1 : Sum  Inputs=+-
  Gain1 : Gain  Gain=exp(-n)
  Transfer Fcn : TransferFcn  Numerator=[W]  Denominator=[1 n/(2*T)]
  Transfer Fcn1 : TransferFcn  Numerator=[W]  Denominator=[1 n/(2*T)]
  Out1 : Outport
  wires:
  In2/1 -> Transfer Fcn1/1
  Gain1/1 -> Add1/2
  In1/1 -> Transfer Fcn/1
  Transfer Fcn/1 -> Add1/1
  Transfer Fcn1/1 -> Gain1/1
  Add1/1 -> Out1/1

== system usask_segmented_TLM_lib/Internal Functions/H/Part 1/Filter4 ==
  In1 : Inport
  In2 : Inport  Port=2
  Add1 : Sum  Inputs=+-
  Gain1 : Gain  Gain=exp(-n)
  Transfer Fcn : TransferFcn  Numerator=[W]  Denominator=[1 n/(2*T)]
  Transfer Fcn1 : TransferFcn  Numerator=[W]  Denominator=[1 n/(2*T)]
  Out1 : Outport
  wires:
  Add1/1 -> Out1/1
  Transfer Fcn1/1 -> Gain1/1
  Transfer Fcn/1 -> Add1/1
  In1/1 -> Transfer Fcn/1
  Gain1/1 -> Add1/2
  In2/1 -> Transfer Fcn1/1

== system usask_segmented_TLM_lib/Internal Functions/H/Part 1/Filter5 ==
  In1 : Inport
  In2 : Inport  Port=2
  Add1 : Sum  Inputs=+-
  Gain1 : Gain  Gain=exp(-n)
  Transfer Fcn : TransferFcn  Numerator=[W]  Denominator=[1 n/(2*T)]
  Transfer Fcn1 : TransferFcn  Numerator=[W]  Denominator=[1 n/(2*T)]
  Out1 : Outport
  wires:
  In2/1 -> Transfer Fcn1/1
  Gain1/1 -> Add1/2
  In1/1 -> Transfer Fcn/1
  Transfer Fcn/1 -> Add1/1
  Transfer Fcn1/1 -> Gain1/1
  Add1/1 -> Out1/1

== system usask_segmented_TLM_lib/Internal Functions/H/Part 1/Filter6 ==
  In1 : Inport
  In2 : Inport  Port=2
  Add1 : Sum  Inputs=+-
  Gain1 : Gain  Gain=exp(-n)
  Transfer Fcn : TransferFcn  Numerator=[W]  Denominator=[1 n/(2*T)]
  Transfer Fcn1 : TransferFcn  Numerator=[W]  Denominator=[1 n/(2*T)]
  Out1 : Outport
  wires:
  Add1/1 -> Out1/1
  Transfer Fcn1/1 -> Gain1/1
  Transfer Fcn/1 -> Add1/1
  In1/1 -> Transfer Fcn/1
  Gain1/1 -> Add1/2
  In2/1 -> Transfer Fcn1/1

== system usask_segmented_TLM_lib/Internal Functions/H/Part 2/Filter1 ==
  In1 : Inport
  In2 : Inport  Port=2
  Add1 : Sum  Inputs=+-
  Gain1 : Gain  Gain=exp(-n)
  Transfer Fcn : TransferFcn  Numerator=[W]  Denominator=[1 n/(2*T)]
  Transfer Fcn1 : TransferFcn  Numerator=[W]  Denominator=[1 n/(2*T)]
  Out1 : Outport
  wires:
  In2/1 -> Transfer Fcn1/1
  Gain1/1 -> Add1/2
  In1/1 -> Transfer Fcn/1
  Transfer Fcn/1 -> Add1/1
  Transfer Fcn1/1 -> Gain1/1
  Add1/1 -> Out1/1

== system usask_segmented_TLM_lib/Internal Functions/H/Part 2/Filter2 ==
  In1 : Inport
  In2 : Inport  Port=2
  Add1 : Sum  Inputs=+-
  Gain1 : Gain  Gain=exp(-n)
  Transfer Fcn : TransferFcn  Numerator=[W]  Denominator=[1 n/(2*T)]
  Transfer Fcn1 : TransferFcn  Numerator=[W]  Denominator=[1 n/(2*T)]
  Out1 : Outport
  wires:
  Add1/1 -> Out1/1
  Transfer Fcn1/1 -> Gain1/1
  Transfer Fcn/1 -> Add1/1
  In1/1 -> Transfer Fcn/1
  Gain1/1 -> Add1/2
  In2/1 -> Transfer Fcn1/1

== system usask_segmented_TLM_lib/Internal Functions/H/Part 2/Filter3 ==
  In1 : Inport
  In2 : Inport  Port=2
  Add1 : Sum  Inputs=+-
  Gain1 : Gain  Gain=exp(-n)
  Transfer Fcn : TransferFcn  Numerator=[W]  Denominator=[1 n/(2*T)]
  Transfer Fcn1 : TransferFcn  Numerator=[W]  Denominator=[1 n/(2*T)]
  Out1 : Outport
  wires:
  In2/1 -> Transfer Fcn1/1
  Gain1/1 -> Add1/2
  In1/1 -> Transfer Fcn/1
  Transfer Fcn/1 -> Add1/1
  Transfer Fcn1/1 -> Gain1/1
  Add1/1 -> Out1/1

== system usask_segmented_TLM_lib/Internal Functions/H/Part 2/Filter4 ==
  In1 : Inport
  In2 : Inport  Port=2
  Add1 : Sum  Inputs=+-
  Gain1 : Gain  Gain=exp(-n)
  Transfer Fcn : TransferFcn  Numerator=[W]  Denominator=[1 n/(2*T)]
  Transfer Fcn1 : TransferFcn  Numerator=[W]  Denominator=[1 n/(2*T)]
  Out1 : Outport
  wires:
  Add1/1 -> Out1/1
  Transfer Fcn1/1 -> Gain1/1
  Transfer Fcn/1 -> Add1/1
  In1/1 -> Transfer Fcn/1
  Gain1/1 -> Add1/2
  In2/1 -> Transfer Fcn1/1

== system usask_segmented_TLM_lib/Internal Functions/H/Part 2/Filter5 ==
  In1 : Inport
  In2 : Inport  Port=2
  Add1 : Sum  Inputs=+-
  Gain1 : Gain  Gain=exp(-n)
  Transfer Fcn : TransferFcn  Numerator=[W]  Denominator=[1 n/(2*T)]
  Transfer Fcn1 : TransferFcn  Numerator=[W]  Denominator=[1 n/(2*T)]
  Out1 : Outport
  wires:
  In2/1 -> Transfer Fcn1/1
  Gain1/1 -> Add1/2
  In1/1 -> Transfer Fcn/1
  Transfer Fcn/1 -> Add1/1
  Transfer Fcn1/1 -> Gain1/1
  Add1/1 -> Out1/1

== system usask_segmented_TLM_lib/Internal Functions/H/Part 2/Filter6 ==
  In1 : Inport
  In2 : Inport  Port=2
  Add1 : Sum  Inputs=+-
  Gain1 : Gain  Gain=exp(-n)
  Transfer Fcn : TransferFcn  Numerator=[W]  Denominator=[1 n/(2*T)]
  Transfer Fcn1 : TransferFcn  Numerator=[W]  Denominator=[1 n/(2*T)]
  Out1 : Outport
  wires:
  Add1/1 -> Out1/1
  Transfer Fcn1/1 -> Gain1/1
  Transfer Fcn/1 -> Add1/1
  In1/1 -> Transfer Fcn/1
  Gain1/1 -> Add1/2
  In2/1 -> Transfer Fcn1/1
